simulink model "RocketStability_ImpulseResponse"  (R2014a)
settings: Solver=ode3  StartTime=0.0  StopTime=25  FixedStep=0.01  MinStep=0.01  RelTol=1e-3
libraries: rocket_angular_flight_library x2, rocket_vertical_flight_library x1
settings Model: Creator=scorpii  LastModifiedBy=scorpii
settings SolverCC: InitialStep=0.01
settings DataIOCC: LimitDataPoints=off
settings OptimizationCC: SimCompilerOptimization=off
settings DebuggingCC: ArtificialAlgebraicLoopMsg=error  MergeDetectMultiDrivingBlocksExec=error  FrameProcessingCompatibilityMsg=error
settings RTWCC: RTWCompilerOptimization=off

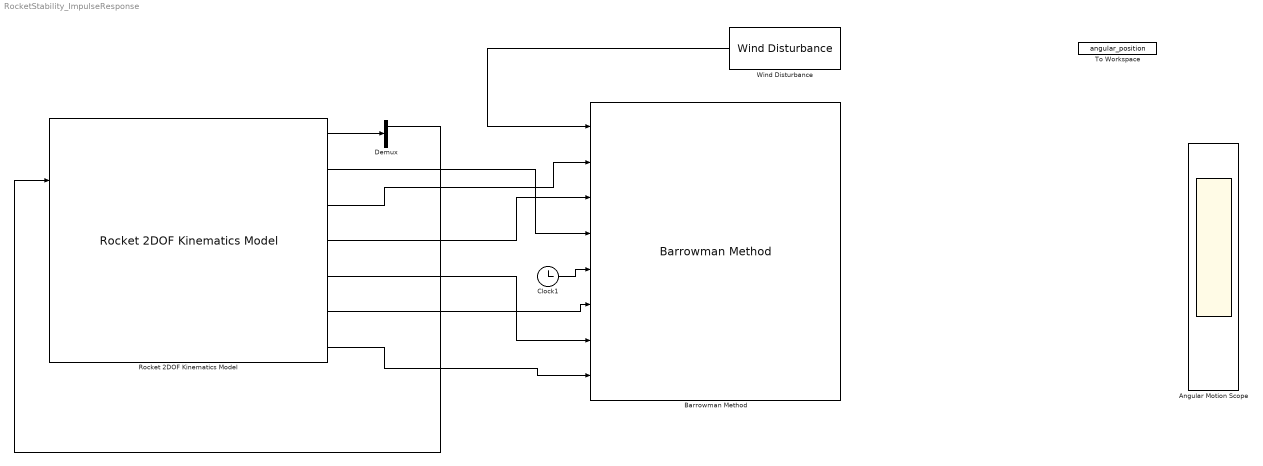
== system RocketStability_ImpulseResponse ==
  Angular Motion Scope : Scope  NumInputPorts=6
      settings: TimeRange=10  YMin=-0.7~-0.125~-0.015~0.05~9~-5  YMax=0.9~0.125~0.015~0.275~24~5  SaveName=ScopeData5
  Barrowman Method : rocket_angular_flight_library/Barrowman Method
  Clock1 : Clock
  Demux : Demux  Outputs=2
  Rocket 2DOF Kinematics Model : rocket_vertical_flight_library/Rocket 2DOF Kinematics Model
  To Workspace : ToWorkspace  VariableName=angular_position  SampleTime=-1
  Wind Disturbance : rocket_angular_flight_library/Wind Disturbance
  wires:
  ? -> Angular Motion Scope/2
  ? -> Angular Motion Scope/1
  Clock1/1 -> Barrowman Method/5
  ? -> Angular Motion Scope/5
  ? -> Angular Motion Scope/4
  ? -> Angular Motion Scope/6
  ? -> Rocket 2DOF Kinematics Model/2
  Demux/1 -> Rocket 2DOF Kinematics Model/1
  Rocket 2DOF Kinematics Model/1 -> Demux/1
  Rocket 2DOF Kinematics Model/2 -> Barrowman Method/4
  Rocket 2DOF Kinematics Model/3 -> Barrowman Method/2
  Rocket 2DOF Kinematics Model/4 -> Barrowman Method/3
  Rocket 2DOF Kinematics Model/5 -> Barrowman Method/7
  Rocket 2DOF Kinematics Model/6 -> Barrowman Method/6
  Rocket 2DOF Kinematics Model/7 -> Barrowman Method/8
  ? -> To Workspace/1, Wind Disturbance/1
  Wind Disturbance/1 -> Barrowman Method/1
